simulink model "kiem_chung_con_lac"  (R2025a)
settings: Solver=ode23  StartTime=0.0  StopTime=5  RelTol=1e-3
values from neighbouring files (symbols this model uses):
  Kdc = 6.52501634734    [PID_con_lac.mat]
  Kic = 98.7160085219    [PID_con_lac.mat]
  Kpc = 50.6645972215    [PID_con_lac.mat]
undefined symbols (not defined in the file or in its folder): G2, impulseAmplitude, impulseDuration
settings Model: Creator=datng  LastModifiedBy=datng

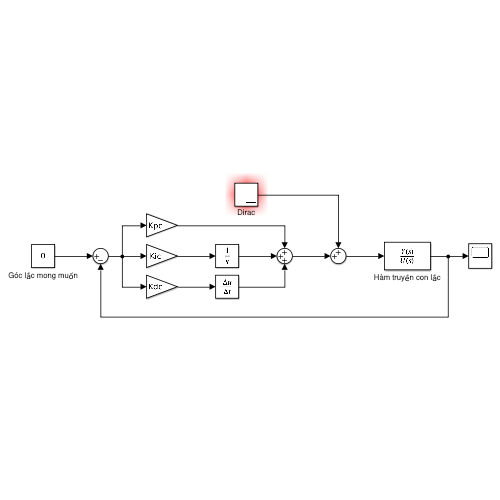
[thumbnail: Simulink's stored preview of the top-level diagram]
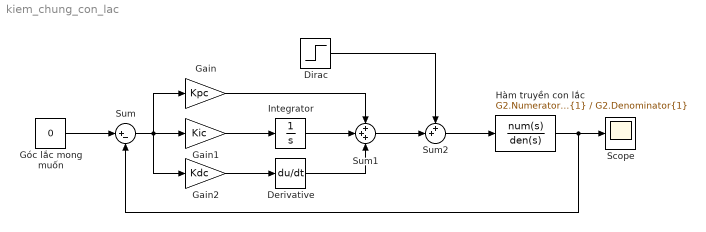
== system kiem_chung_con_lac ==
  Derivative : Derivative  CoefficientInTFapproximation=0
  Dirac : Step  Time=impulseDuration  Before=impulseAmplitude  After=0  SampleTime=0
  Gain : Gain  Gain=Kpc
  Gain1 : Gain  Gain=Kic
  Gain2 : Gain  Gain=Kdc
  Góc lắc mong muốn : Constant  Value=0
  Hàm truyền con lắc : TransferFcn  Numerator=G2.Numerator{1}  Denominator=G2.Denominator{1}
  Integrator : Integrator
  Scope : Scope
      settings: ActiveDisplayYMinimum=-0.008764263071145471  ActiveDisplayYMaximum=0.0489006906512177
  Sum : Sum  Inputs=|+-
  Sum1 : Sum  Inputs=+++
  Sum2 : Sum  Inputs=++|
  wires:
  Góc lắc mong muốn/1 -> Sum/1
  Sum/1 -> Gain/1, Gain2/1, Gain1/1
  Gain1/1 -> Integrator/1
  Integrator/1 -> Sum1/2
  Derivative/1 -> Sum1/3
  Gain2/1 -> Derivative/1
  Gain/1 -> Sum1/1
  Sum1/1 -> Sum2/2
  Dirac/1 -> Sum2/1
  Sum2/1 -> Hàm truyền con lắc/1
  Hàm truyền con lắc/1 -> Sum/2, Scope/1
